simulink model "schema_alocare_testare_numerica"  (R2023a)
settings: Solver=VariableStepAuto  StartTime=0.0  StopTime=20  RelTol=1e-3
values from neighbouring files (symbols this model uses):
  Ts = 0.2    [Untitled.m]
undefined symbols (not defined in the file or in its folder): den0z, den1pz, denr_s, num0z, num1pz, numr_s
settings Model: Creator=Traxar72  LastModifiedBy=Traxar72

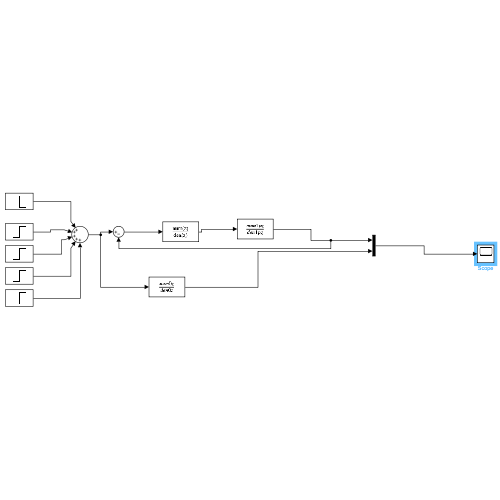
[thumbnail: Simulink's stored preview of the top-level diagram]
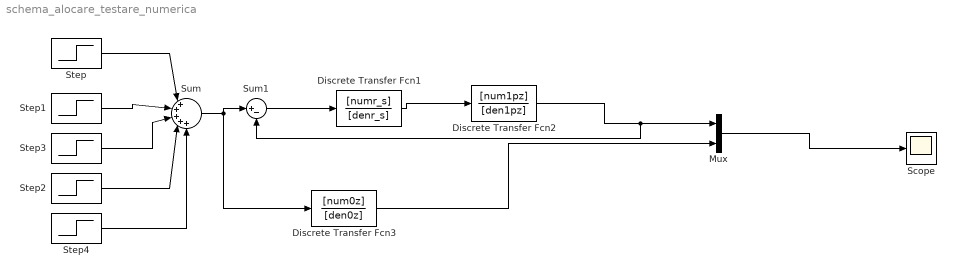
== system schema_alocare_testare_numerica ==
  Discrete Transfer Fcn1 : DiscreteTransferFcn  Numerator=[numr_s]  Denominator=[denr_s]  SampleTime=Ts
  Discrete Transfer Fcn2 : DiscreteTransferFcn  Numerator=[num1pz]  Denominator=[den1pz]  SampleTime=Ts
  Discrete Transfer Fcn3 : DiscreteTransferFcn  Numerator=[num0z]  Denominator=[den0z]  SampleTime=Ts
  Mux : Mux  Inputs=2
  Scope : Scope
  Step : Step  Time=16  After=-4  SampleTime=Ts
  Step1 : Step  Time=12  SampleTime=Ts
  Step2 : Step  Time=4  SampleTime=Ts
  Step3 : Step  Time=8  SampleTime=Ts
  Step4 : Step  Time=0  SampleTime=Ts
  Sum : Sum  Inputs=|+++++
  Sum1 : Sum  Inputs=|+-
  wires:
  Discrete Transfer Fcn2/1 -> Sum1/2, Mux/1
  Discrete Transfer Fcn1/1 -> Discrete Transfer Fcn2/1
  Sum1/1 -> Discrete Transfer Fcn1/1
  Discrete Transfer Fcn3/1 -> Mux/2
  Step4/1 -> Sum/5
  Mux/1 -> Scope/1
  Step2/1 -> Sum/4
  Sum/1 -> Discrete Transfer Fcn3/1, Sum1/1
  Step3/1 -> Sum/3
  Step1/1 -> Sum/2
  Step/1 -> Sum/1
